simulink model "Capstone_30V_Prototype"  (R2025a)
settings: Solver=VariableStepAuto  StartTime=0.0  StopTime=1.0  RelTol=1e-3
libraries: spsCurrentMeasurementLib x5, spsSeriesRLCBranchLib x5, spsVoltageMeasurementLib x4, spsACVoltageSourceLib x1, sps_lib x1
settings Model: Creator=jamesthompson  LastModifiedBy=jamesthompson

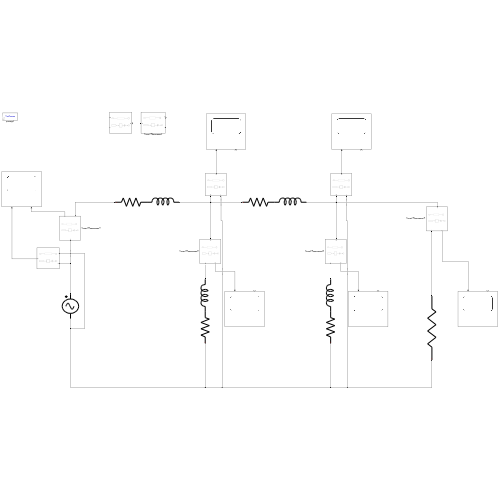
[thumbnail: Simulink's stored preview of the top-level diagram]
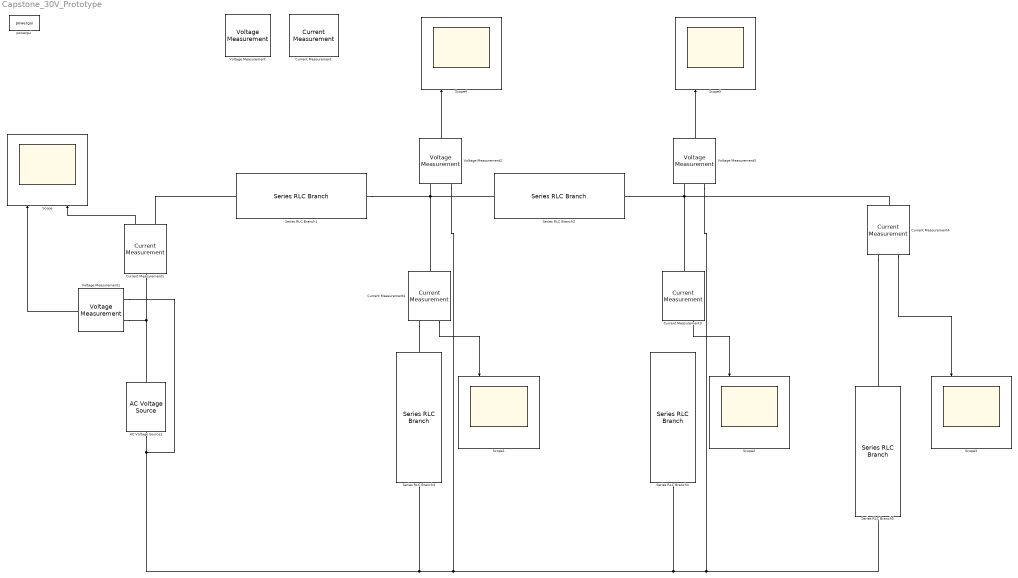
== system Capstone_30V_Prototype ==
  AC Voltage Source1 : spsACVoltageSourceLib/AC Voltage Source  Amplitude=42.43  Phase=0  Frequency=60  SampleTime=0  Measurements=None  BusType=swing  Pref=10e3  Qref=0  Qmin=-inf  Qmax=+inf
  Current Measurement{,1..4} (5 alike) : spsCurrentMeasurementLib/Current Measurement  PhasorSimulation=off  OutputType=Complex  PSBequivalent=0
  Scope{,1..5} (6 alike) : Scope  NumInputPorts=2
      Scope settings: ActiveDisplayYMinimum=-53.037499597731021  ActiveDisplayYMaximum=53.037499701417083
      Scope1 settings: ActiveDisplayYMinimum=-5.5490592381946069  ActiveDisplayYMaximum=5.5490601629731389
      Scope2 settings: ActiveDisplayYMinimum=-1  ActiveDisplayYMaximum=1  DataLoggingVariableName=ScopeData2
      Scope3 settings: ActiveDisplayYMinimum=-4.4848631924562126  ActiveDisplayYMaximum=4.4893069116132738  DataLoggingVariableName=ScopeData3
      Scope4 settings: ActiveDisplayYMinimum=1.5752101789756709  ActiveDisplayYMaximum=1.6367751879799648  DataLoggingVariableName=ScopeData4
      Scope5 settings: ActiveDisplayYMinimum=-44.848631924562113  ActiveDisplayYMaximum=44.893069116132729  DataLoggingVariableName=ScopeData5
  Series RLC Branch1 : spsSeriesRLCBranchLib/Series RLC Branch  LConnTagsString=__new0  RConnTagsString=__new0  BranchType=RL  Resistance=1  Inductance=0.9e-6  SetiL0=off  InitialCurrent=0  Capacitance=1e-6  Setx0=off  InitialVoltage=0  Measurements=None
  Series RLC Branch2 : spsSeriesRLCBranchLib/Series RLC Branch  LConnTagsString=__new0  RConnTagsString=__new0  BranchType=RL  Resistance=0.5  Inductance=0.1e-3  SetiL0=off  InitialCurrent=0  Capacitance=1e-6  Setx0=off  InitialVoltage=0  Measurements=None
  Series RLC Branch3 : spsSeriesRLCBranchLib/Series RLC Branch  LConnTagsString=__new0  RConnTagsString=__new0  BranchType=RL  Resistance=1.8  Inductance=22e-3  SetiL0=off  InitialCurrent=0  Capacitance=1e-6  Setx0=off  InitialVoltage=0  Measurements=None
  Series RLC Branch4 : spsSeriesRLCBranchLib/Series RLC Branch  LConnTagsString=__new0  RConnTagsString=__new0  BranchType=RL  Resistance=1.8  Inductance=22e-3  SetiL0=off  InitialCurrent=0  Capacitance=1e-6  Setx0=off  InitialVoltage=0  Measurements=None
  Series RLC Branch5 : spsSeriesRLCBranchLib/Series RLC Branch  LConnTagsString=__new0  RConnTagsString=__new0  BranchType=R  Resistance=10  Inductance=1e-3  SetiL0=off  InitialCurrent=0  Capacitance=1e-6  Setx0=off  InitialVoltage=0  Measurements=None
  Voltage Measurement{,1..3} (4 alike) : spsVoltageMeasurementLib/Voltage Measurement  PhasorSimulation=off  OutputType=Complex  PSBequivalent=0
  powergui : sps_lib/powergui  Priority=1  SimulationMode=Continuous  SampleTime=50e-6  frequency=60  Iterations=50  frequencyindice=60  Pbase=100e6  ErrMax=1e-4  UnitsV=kV  UnitsW=MW  buscounter=0  FunctionMessages=off  echomessages=off  EnableUseOfTLC=off  CurrentSourceSwitches=off  DisableSnubberDevices=off  DisableRonSwitches=off  DisableVfSwitches=off  DisplayEquations=off  AutomaticDiscreteSolvers=off  SolverType=Tustin/Backward Euler (TBE)  Interpol=off  ExternalGateDelay=off  methode=off  Ts=100  x0status=blocks  SPID=on  SwTol=0  HookPort=off  NonlinearTolerance=1e-4  nMaxIteration=100  ContinueOnMaxIteration=off  RestoreLinks=warning  ResistiveCurrentMeasurement=off  Frange=[0:2:500]  Ylog=off  Xlog=on  ShowGrid=off  save=off  variable=ZData  structure=0  ZoomFFT=off  StartTime=0.0  cycles=1  DisplayStyle=1  fundamental=60  FreqAxis=off  MaxFrequency=1000  frequencyindicesteady=1  RmsSteady=1  display=off
  wires:
  Current Measurement1/1 -> Scope/2
  Voltage Measurement1/1 -> Scope/1
  Current Measurement2/1 -> Scope1/1
  Current Measurement3/1 -> Scope2/1
  Current Measurement4/1 -> Scope3/1
  Voltage Measurement2/1 -> Scope4/1
  Voltage Measurement3/1 -> Scope5/1
  connections:
  Current Measurement1/RConn1 -- Series RLC Branch1/LConn1
  Series RLC Branch1/RConn1 -- Series RLC Branch2/LConn1 -- Current Measurement2/LConn1 -- Voltage Measurement2/LConn1
  Series RLC Branch2/RConn1 -- Current Measurement4/LConn1 -- Voltage Measurement3/LConn1 -- Current Measurement3/LConn1
  Current Measurement4/RConn1 -- Series RLC Branch5/RConn1
  AC Voltage Source1/LConn1 -- Voltage Measurement1/LConn2 -- Series RLC Branch3/LConn1 -- Voltage Measurement2/LConn2 -- Series RLC Branch4/LConn1 -- Voltage Measurement3/LConn2 -- Series RLC Branch5/LConn1
  Current Measurement1/LConn1 -- Voltage Measurement1/LConn1 -- AC Voltage Source1/RConn1
  Current Measurement2/RConn1 -- Series RLC Branch3/RConn1
